simulink library "CTRL"  (R2024b)
settings: Solver=VariableStepAuto  StartTime=0.0  StopTime=10.0  RelTol=1e-3
libraries: simulink x2, CTRL_BASECTRL x1, CTRL_FUS x1, CTRL_SPECCTRL x1
settings Model: Creator=blatak  LastModifiedBy=blatak
settings ModelReferenceCC: EnableRefExpFcnMdlSchedulingChecks=on
settings RTWCC: GPUComputeCapability=3.5

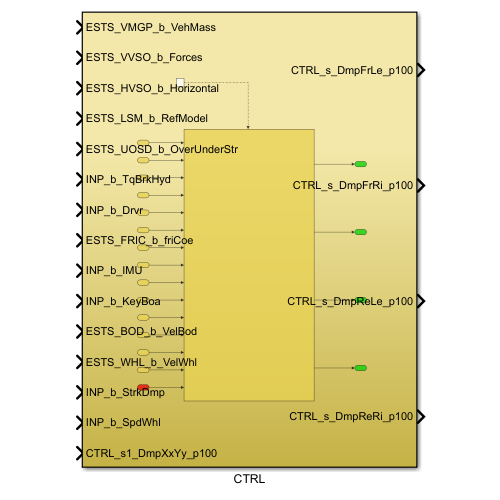
[thumbnail: Simulink's stored preview of the top-level diagram]
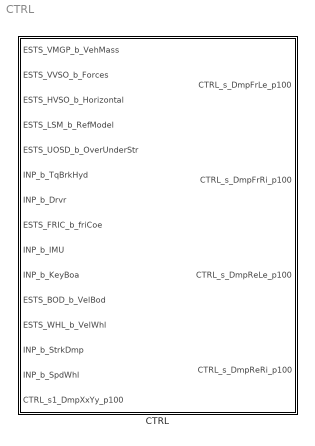
== system CTRL ==
  CTRL : Subsystem

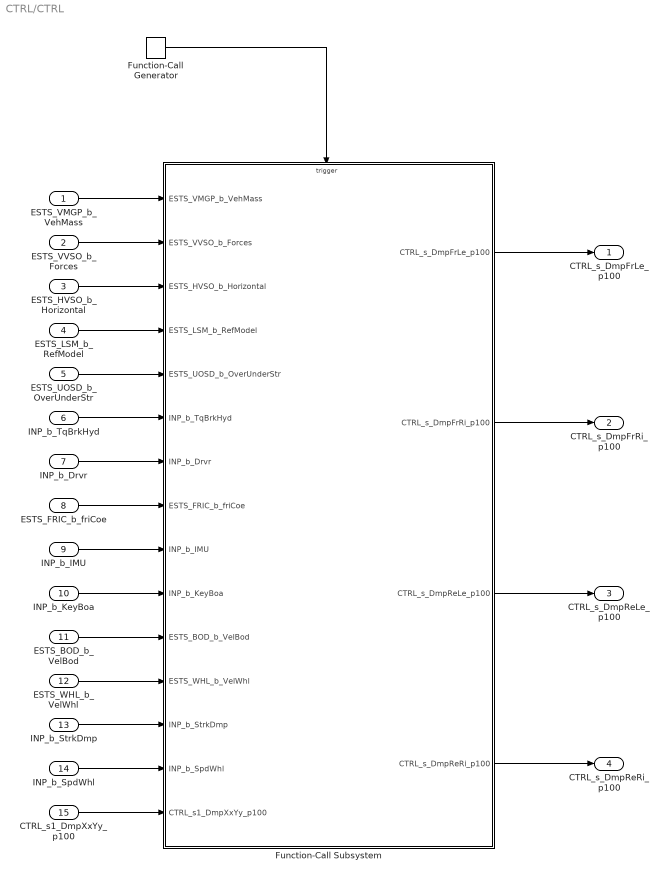
== system CTRL/CTRL ==
  ESTS_VMGP_b_VehMass : Inport
  ESTS_VVSO_b_Forces : Inport  Port=2
  ESTS_HVSO_b_Horizontal : Inport  Port=3
  ESTS_LSM_b_RefModel : Inport  Port=4
  ESTS_UOSD_b_OverUnderStr : Inport  Port=5
  INP_b_TqBrkHyd : Inport  Port=6
  INP_b_Drvr : Inport  Port=7
  ESTS_FRIC_b_friCoe : Inport  Port=8
  INP_b_IMU : Inport  Port=9
  INP_b_KeyBoa : Inport  Port=10
  ESTS_BOD_b_VelBod : Inport  Port=11
  ESTS_WHL_b_VelWhl : Inport  Port=12
  INP_b_StrkDmp : Inport  Port=13
  INP_b_SpdWhl : Inport  Port=14
  CTRL_s1_DmpXxYy_p100 : Inport  Port=15
  Function-Call Generator : simulink/Ports & Subsystems/Function-Call Generator  sample_time=0.005  numberOfIterations=1  DisallowWideOutput=off
  Function-Call Subsystem : Subsystem  TreatAsAtomicUnit=on
  CTRL_s_DmpFrLe_p100 : Outport
  CTRL_s_DmpFrRi_p100 : Outport  Port=2
  CTRL_s_DmpReLe_p100 : Outport  Port=3
  CTRL_s_DmpReRi_p100 : Outport  Port=4
  wires:
  Function-Call Generator/1 -> Function-Call Subsystem/Trigger
  ESTS_VMGP_b_VehMass/1 -> Function-Call Subsystem/1(ESTS_VMGP_b_VehMass)
  ESTS_VVSO_b_Forces/1 -> Function-Call Subsystem/2(ESTS_VVSO_b_Forces)
  ESTS_HVSO_b_Horizontal/1 -> Function-Call Subsystem/3(ESTS_HVSO_b_Horizontal)
  ESTS_LSM_b_RefModel/1 -> Function-Call Subsystem/4(ESTS_LSM_b_RefModel)
  ESTS_UOSD_b_OverUnderStr/1 -> Function-Call Subsystem/5(ESTS_UOSD_b_OverUnderStr)
  INP_b_TqBrkHyd/1 -> Function-Call Subsystem/6(INP_b_TqBrkHyd)
  INP_b_Drvr/1 -> Function-Call Subsystem/7(INP_b_Drvr)
  ESTS_FRIC_b_friCoe/1 -> Function-Call Subsystem/8(ESTS_FRIC_b_friCoe)
  INP_b_IMU/1 -> Function-Call Subsystem/9(INP_b_IMU)
  INP_b_KeyBoa/1 -> Function-Call Subsystem/10(INP_b_KeyBoa)
  Function-Call Subsystem/1(CTRL_s_DmpFrLe_p100) -> CTRL_s_DmpFrLe_p100/1
  Function-Call Subsystem/2(CTRL_s_DmpFrRi_p100) -> CTRL_s_DmpFrRi_p100/1
  Function-Call Subsystem/3(CTRL_s_DmpReLe_p100) -> CTRL_s_DmpReLe_p100/1
  Function-Call Subsystem/4(CTRL_s_DmpReRi_p100) -> CTRL_s_DmpReRi_p100/1
  ESTS_BOD_b_VelBod/1 -> Function-Call Subsystem/11(ESTS_BOD_b_VelBod)
  ESTS_WHL_b_VelWhl/1 -> Function-Call Subsystem/12(ESTS_WHL_b_VelWhl)
  INP_b_StrkDmp/1 -> Function-Call Subsystem/13(INP_b_StrkDmp)
  INP_b_SpdWhl/1 -> Function-Call Subsystem/14(INP_b_SpdWhl)
  CTRL_s1_DmpXxYy_p100/1 -> Function-Call Subsystem/15(CTRL_s1_DmpXxYy_p100)

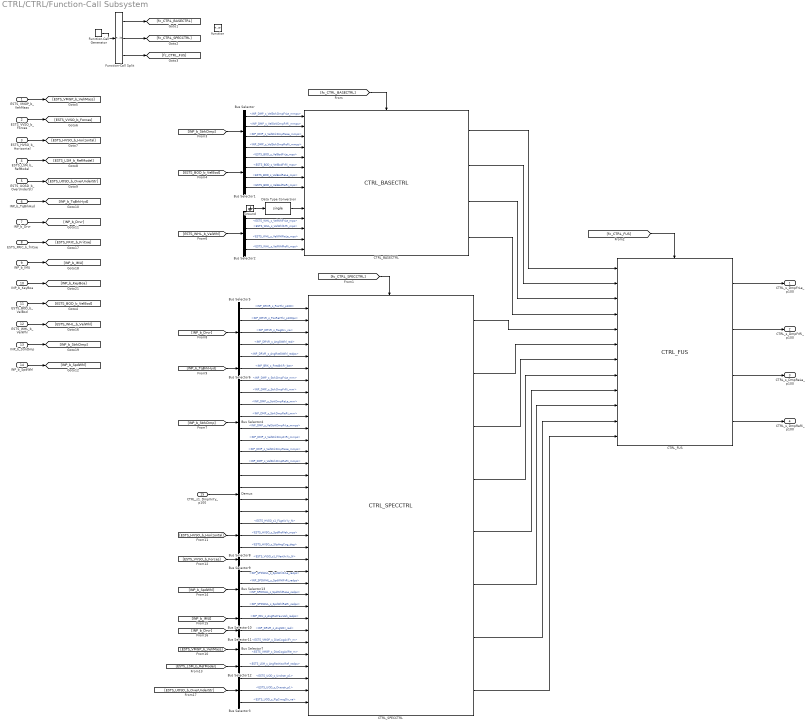
== system CTRL/CTRL/Function-Call Subsystem ==
  ESTS_VMGP_b_VehMass : Inport
  ESTS_VVSO_b_Forces : Inport  Port=2
  ESTS_HVSO_b_Horizontal : Inport  Port=3
  ESTS_LSM_b_RefModel : Inport  Port=4
  ESTS_UOSD_b_OverUnderStr : Inport  Port=5
  INP_b_TqBrkHyd : Inport  Port=6
  INP_b_Drvr : Inport  Port=7
  ESTS_FRIC_b_friCoe : Inport  Port=8
  INP_b_IMU : Inport  Port=9
  INP_b_KeyBoa : Inport  Port=10
  ESTS_BOD_b_VelBod : Inport  Port=11
  ESTS_WHL_b_VelWhl : Inport  Port=12
  INP_b_StrkDmp : Inport  Port=13
  INP_b_SpdWhl : Inport  Port=14
  CTRL_s1_DmpXxYy_p100 : Inport  Port=15
  function : TriggerPort  TriggerType=function-call  VariantControl=(inherit)
  Bus Selector : BusSelector  OutputSignals=INP_DMP_s_VelStrkDmpFrLe_mmps,INP_DMP_s_VelStrkDmpFrRi_mmps,INP_DMP_s_VelStrkDmpReLe_mmps,INP_DMP_s_VelStrkDmpReRi_mmps
  Bus Selector1 : BusSelector  OutputSignals=ESTS_BOD_s_VelBodFrLe_mps,ESTS_BOD_s_VelBodFrRi_mps,ESTS_BOD_s_VelBodReLe_mps,ESTS_BOD_s_VelBodReRi_mps
  Bus Selector10 : BusSelector  OutputSignals=INP_IMU_s_AngRatYawVeh_radps
  Bus Selector11 : BusSelector  OutputSignals=INP_DRVR_s_AngStFr_rad
  Bus Selector12 : BusSelector  OutputSignals=ESTS_LSM_s_AngRatYawRef_radps
  Bus Selector13 : BusSelector  OutputSignals=INP_SPDWHL_s_SpdWhlFrLe_radps,INP_SPDWHL_s_SpdWhlFrRi_radps,INP_SPDWHL_s_SpdWhlReLe_radps,INP_SPDWHL_s_SpdWhlReRi_radps
  Bus Selector2 : BusSelector  OutputSignals=ESTS_WHL_s_VelWhlFrLe_mps,ESTS_WHL_s_VelWhlFrRi_mps,ESTS_WHL_s_VelWhlReLe_mps,ESTS_WHL_s_VelWhlReRi_mps
  Bus Selector3 : BusSelector  OutputSignals=ESTS_UOD_s_Undrstr_p1,ESTS_UOD_s_Overstr_p1,ESTS_UOD_s_FlgCrnrgDir_na
  Bus Selector4 : BusSelector  OutputSignals=INP_DMP_s_StrkDmpFrLe_mm,INP_DMP_s_StrkDmpFrRi_mm,INP_DMP_s_StrkDmpReLe_mm,INP_DMP_s_StrkDmpReRi_mm,INP_DMP_s_VelStrkDmpFrLe_mmps,INP_DMP_s_VelStrkDmpFrRi_mmps,INP_DMP_s_VelStrkDmpReLe_mmps,INP_DMP_s_VelStrkDmpReRi_mmps
  Bus Selector5 : BusSelector  OutputSignals=INP_DRVR_s_PosThr_p100,INP_DRVR_s_PosRatThr_p100ps,INP_DRVR_s_RegDrv_na,INP_DRVR_s_AngStWhl_rad,INP_DRVR_s_AngRatStWhl_radps
  Bus Selector6 : BusSelector  OutputSignals=INP_BRK_s_PresBrkFr_bar
  Bus Selector7 : BusSelector  OutputSignals=ESTS_VMGP_s_DistCogAxlFr_m,ESTS_VMGP_s_DistCogAxlRe_m
  Bus Selector8 : BusSelector  OutputSignals=ESTS_HVSO_s1_FLgtXxYy_N,ESTS_HVSO_s_SpdRefVeh_mps,ESTS_HVSO_s_SlipAngCog_deg
  Bus Selector9 : BusSelector  OutputSignals=ESTS_VVSO_s1_FVertXxYy_N
  CTRL_BASECTRL : CTRL_BASECTRL/CTRL_BASECTRL  SystemSampleTime=-1  VariantActivationTime=update diagram  AllowFlexibleInterface=on  Latency=0  AutoFrameSizeCalculation=off
  CTRL_FUS : CTRL_FUS/CTRL_FUS  SystemSampleTime=-1  VariantActivationTime=update diagram  AllowFlexibleInterface=on  Latency=0  AutoFrameSizeCalculation=off
  CTRL_SPECCTRL : CTRL_SPECCTRL/CTRL_SPECCTRL  SystemSampleTime=-1  VariantActivationTime=update diagram  AllowFlexibleInterface=on  Latency=0  AutoFrameSizeCalculation=off
  Data Type Conversion : DataTypeConversion  OutDataTypeStr=single  SaturateOnIntegerOverflow=off  RndMeth=Floor
  Demux : Demux
  Function-Call Generator : simulink/Ports & Subsystems/Function-Call Generator  sample_time=-1  numberOfIterations=1  DisallowWideOutput=off
  Function-Call Split : FunctionCallSplit  IconShape=distinctive  NumOutputPorts=3  OutputPortLayout=default
  Ground : Ground
  CTRL_s_DmpFrLe_p100 : Outport
  CTRL_s_DmpFrRi_p100 : Outport  Port=2
  CTRL_s_DmpReLe_p100 : Outport  Port=3
  CTRL_s_DmpReRi_p100 : Outport  Port=4
  wires:
  Function-Call Generator/1 -> Function-Call Split/1
  Function-Call Split/1 -> [fc_CTRL_BASECTRL]
  Function-Call Split/2 -> [fc_CTRL_SPECCTRL]
  Function-Call Split/3 -> [fc_CTRL_FUS]
  ESTS_VMGP_b_VehMass/1 -> [ESTS_VMGP_b_VehMass]
  INP_b_Drvr/1 -> [INP_b_Drvr]
  INP_b_TqBrkHyd/1 -> [INP_b_TqBrkHyd]
  ESTS_UOSD_b_OverUnderStr/1 -> [ESTS_UOSD_b_OverUnderStr]
  ESTS_LSM_b_RefModel/1 -> [ESTS_LSM_b_RefModel]
  ESTS_HVSO_b_Horizontal/1 -> [ESTS_HVSO_b_Horizontal]
  ESTS_VVSO_b_Forces/1 -> [ESTS_VVSO_b_Forces]
  ESTS_FRIC_b_friCoe/1 -> [ESTS_FRIC_b_FriCoe]
  INP_b_IMU/1 -> [INP_b_IMU]
  INP_b_KeyBoa/1 -> [INP_b_KeyBoa]
  [fc_CTRL_BASECTRL] -> CTRL_BASECTRL/Trigger
  [fc_CTRL_SPECCTRL] -> CTRL_SPECCTRL/Trigger
  [fc_CTRL_FUS] -> CTRL_FUS/Trigger
  ESTS_BOD_b_VelBod/1 -> [ESTS_BOD_b_VelBod]
  ESTS_WHL_b_VelWhl/1 -> [ESTS_WHL_b_VelWhl]
  INP_b_StrkDmp/1 -> [INP_b_StrkDmp]
  [INP_b_StrkDmp] -> Bus Selector/1
  Bus Selector/1 -> CTRL_BASECTRL/1  "<INP_DMP_s_VelStrkDmpFrLe_mmps>"
  Bus Selector/2 -> CTRL_BASECTRL/2  "<INP_DMP_s_VelStrkDmpFrRi_mmps>"
  Bus Selector/3 -> CTRL_BASECTRL/3  "<INP_DMP_s_VelStrkDmpReLe_mmps>"
  Bus Selector/4 -> CTRL_BASECTRL/4  "<INP_DMP_s_VelStrkDmpReRi_mmps>"
  Bus Selector1/1 -> CTRL_BASECTRL/5  "<ESTS_BOD_s_VelBodFrLe_mps>"
  Bus Selector1/2 -> CTRL_BASECTRL/6  "<ESTS_BOD_s_VelBodFrRi_mps>"
  Bus Selector1/3 -> CTRL_BASECTRL/7  "<ESTS_BOD_s_VelBodReLe_mps>"
  Bus Selector1/4 -> CTRL_BASECTRL/8  "<ESTS_BOD_s_VelBodReRi_mps>"
  [ESTS_BOD_b_VelBod] -> Bus Selector1/1
  Bus Selector2/1 -> CTRL_BASECTRL/11  "<ESTS_WHL_s_VelWhlFrLe_mps>"
  Bus Selector2/2 -> CTRL_BASECTRL/12  "<ESTS_WHL_s_VelWhlFrRi_mps>"
  Bus Selector2/3 -> CTRL_BASECTRL/13  "<ESTS_WHL_s_VelWhlReLe_mps>"
  Bus Selector2/4 -> CTRL_BASECTRL/14  "<ESTS_WHL_s_VelWhlReRi_mps>"
  [ESTS_WHL_b_VelWhl] -> Bus Selector2/1
  Data Type Conversion/1 -> CTRL_BASECTRL/10
  Ground/1 -> Data Type Conversion/1
  [INP_b_StrkDmp] -> Bus Selector4/1
  Bus Selector4/1 -> CTRL_SPECCTRL/7  "<INP_DMP_s_StrkDmpFrLe_mm>"
  Bus Selector4/6 -> CTRL_SPECCTRL/12  "<INP_DMP_s_VelStrkDmpFrRi_mmps>"
  Bus Selector4/7 -> CTRL_SPECCTRL/13  "<INP_DMP_s_VelStrkDmpReLe_mmps>"
  Bus Selector4/8 -> CTRL_SPECCTRL/14  "<INP_DMP_s_VelStrkDmpReRi_mmps>"
  Bus Selector4/5 -> CTRL_SPECCTRL/11  "<INP_DMP_s_VelStrkDmpFrLe_mmps>"
  Bus Selector4/2 -> CTRL_SPECCTRL/8  "<INP_DMP_s_StrkDmpFrRi_mm>"
  Bus Selector4/3 -> CTRL_SPECCTRL/9  "<INP_DMP_s_StrkDmpReLe_mm>"
  Bus Selector4/4 -> CTRL_SPECCTRL/10  "<INP_DMP_s_StrkDmpReRi_mm>"
  Bus Selector5/1 -> CTRL_SPECCTRL/1  "<INP_DRVR_s_PosThr_p100>"
  Bus Selector5/2 -> CTRL_SPECCTRL/2  "<INP_DRVR_s_PosRatThr_p100ps>"
  Bus Selector5/4 -> CTRL_SPECCTRL/4  "<INP_DRVR_s_AngStWhl_rad>"
  Bus Selector5/5 -> CTRL_SPECCTRL/5  "<INP_DRVR_s_AngRatStWhl_radps>"
  [INP_b_Drvr] -> Bus Selector5/1
  [INP_b_TqBrkHyd] -> Bus Selector6/1
  Bus Selector6/1 -> CTRL_SPECCTRL/6  "<INP_BRK_s_PresBrkFr_bar>"
  CTRL_BASECTRL/1 -> CTRL_FUS/1
  CTRL_BASECTRL/2 -> CTRL_FUS/2
  CTRL_BASECTRL/3 -> CTRL_FUS/3
  CTRL_BASECTRL/4 -> CTRL_FUS/4
  CTRL_SPECCTRL/1 -> CTRL_FUS/5
  CTRL_SPECCTRL/2 -> CTRL_FUS/6
  CTRL_SPECCTRL/3 -> CTRL_FUS/7
  CTRL_SPECCTRL/4 -> CTRL_FUS/8
  CTRL_SPECCTRL/5 -> CTRL_FUS/9
  CTRL_FUS/1 -> CTRL_s_DmpFrLe_p100/1
  CTRL_FUS/2 -> CTRL_s_DmpFrRi_p100/1
  CTRL_FUS/3 -> CTRL_s_DmpReLe_p100/1
  CTRL_FUS/4 -> CTRL_s_DmpReRi_p100/1
  Bus Selector5/3 -> CTRL_SPECCTRL/3  "<INP_DRVR_s_RegDrv_na>"
  CTRL_s1_DmpXxYy_p100/1 -> Demux/1
  Demux/1 -> CTRL_SPECCTRL/15
  Demux/2 -> CTRL_SPECCTRL/16
  Demux/3 -> CTRL_SPECCTRL/17
  Demux/4 -> CTRL_SPECCTRL/18
  Bus Selector7/1 -> CTRL_SPECCTRL/29  "<ESTS_VMGP_s_DistCogAxlFr_m>"
  Bus Selector7/2 -> CTRL_SPECCTRL/30  "<ESTS_VMGP_s_DistCogAxlRe_m>"
  [ESTS_VMGP_b_VehMass] -> Bus Selector7/1
  Bus Selector8/1 -> CTRL_SPECCTRL/19  "<ESTS_HVSO_s1_FLgtXxYy_N>"
  Bus Selector8/2 -> CTRL_SPECCTRL/20  "<ESTS_HVSO_s_SpdRefVeh_mps>"
  Bus Selector9/1 -> CTRL_SPECCTRL/22  "<ESTS_VVSO_s1_FVertXxYy_N>"
  [ESTS_HVSO_b_Horizontal] -> Bus Selector8/1
  [ESTS_VVSO_b_Forces] -> Bus Selector9/1
  Bus Selector10/1 -> CTRL_SPECCTRL/27  "<INP_IMU_s_AngRatYawVeh_radps>"
  Bus Selector11/1 -> CTRL_SPECCTRL/28  "<INP_DRVR_s_AngStFr_rad>"
  INP_b_SpdWhl/1 -> [INP_b_SpdWhl]
  Bus Selector12/1 -> CTRL_SPECCTRL/31  "<ESTS_LSM_s_AngRatYawRef_radps>"
  [ESTS_LSM_b_RefModel] -> Bus Selector12/1
  Bus Selector13/1 -> CTRL_SPECCTRL/23  "<INP_SPDWHL_s_SpdWhlFrLe_radps>"
  Bus Selector13/2 -> CTRL_SPECCTRL/24  "<INP_SPDWHL_s_SpdWhlFrRi_radps>"
  Bus Selector13/3 -> CTRL_SPECCTRL/25  "<INP_SPDWHL_s_SpdWhlReLe_radps>"
  Bus Selector13/4 -> CTRL_SPECCTRL/26  "<INP_SPDWHL_s_SpdWhlReRi_radps>"
  [INP_b_SpdWhl] -> Bus Selector13/1
  [INP_b_IMU] -> Bus Selector10/1
  [INP_b_Drvr] -> Bus Selector11/1
  Bus Selector8/3 -> CTRL_SPECCTRL/21  "<ESTS_HVSO_s_SlipAngCog_deg>"
  CTRL_SPECCTRL/6 -> CTRL_FUS/10
  CTRL_SPECCTRL/7 -> CTRL_FUS/11
  CTRL_SPECCTRL/8 -> CTRL_FUS/12
  [ESTS_UOSD_b_OverUnderStr] -> Bus Selector3/1
  Bus Selector3/3 -> CTRL_SPECCTRL/34  "<ESTS_UOD_s_FlgCrnrgDir_na>"
  Bus Selector3/2 -> CTRL_SPECCTRL/33  "<ESTS_UOD_s_Overstr_p1>"
  Bus Selector3/1 -> CTRL_SPECCTRL/32  "<ESTS_UOD_s_Undrstr_p1>"
